simulink model "TV_2018_HIL"  (R2016a)
settings: Solver=FixedStepAuto  StartTime=0.0  StopTime=inf  FixedStep=0.001  RelTol=1e-3
PreLoadFcn:
  | TV_2017_parameters
values from neighbouring files (symbols this model uses):
  battery_voltage = single(530)    [HIL_parameters.m]    (also in HIL_parameters_2018.m; TV_2017_parameters.m; TV_2017_parameters_VD.m)
  car_params = Simulink_Car_params    [HIL_parameters.m]    (also in HIL_parameters_2018.m; TV_2017_parameters.m; TV_2017_parameters_VD.m)
  i_Diff = 16    [HIL_parameters.m]    (also in HIL_parameters_2018.m; TV_2017_parameters.m)
  Kp = 1    [HIL_parameters.m]    (also in HIL_parameters_2018.m; TV_2017_parameters.m; TV_2017_parameters_VD.m)
  motor_data = struct    [HIL_parameters.m]    (also in HIL_parameters_2018.m; TV_2017_parameters.m)
  powerLimitControl = Simulink_el    [HIL_parameters.m]    (also in HIL_parameters_2018.m; TV_2017_parameters.m; TV_2017_parameters_VD.m)
  settings = Simulink_Settings    [HIL_parameters.m]    (also in HIL_parameters_2018.m; TV_2017_parameters.m; TV_2017_parameters_VD.m)
  SpdC_BCC = 0    [HIL_parameters.m]    (also in HIL_parameters_2018.m; TV_2017_parameters.m; TV_2017_parameters_VD.m)
  Speed_Neg_sat = -21    [HIL_parameters.m]    (also in HIL_parameters_2018.m; TV_2017_parameters.m; TV_2017_parameters_VD.m)
  Speed_Pos_sat = 21    [HIL_parameters.m]    (also in HIL_parameters_2018.m; TV_2017_parameters.m; TV_2017_parameters_VD.m)
  SteeringAngleFL = [-23.80 -22.65 -21.50 -20.34 -19.18 -18.03 -16.86 -15.70 -14.53 -13.35 -12.18 -10.99 -9.80 -8.61 -7.40 -6.19 -4.97 -3.75 -2.51 -1.26 0 1.27 2.56 3.85 5.17 6.50 7.84 9.21 10.59 12.00 13.42 14.88 16.36 17.87 19.41 20.99 22.61 24.26 25.97 27.73 29.54]    [CarSetupAnalysis2018.m]    (also in HIL_parameters_2018.m; TV_2017_parameters.m; TV_2017_parameters_VD.m = [-24.129 -22.950 -21.772 -20.593 -19.413 -18.232 -17.050 -15)
  SteeringAngleFR = [-29.54 -27.73 -25.97 -24.26 -22.61 -20.99 -19.41 -17.87 -16.36 -14.88 -13.42 -12.00 -10.59 -9.21 -7.84 -6.50 -5.17 -3.85 -2.56 -1.27 0 1.26 2.51 3.75 4.97 6.19 7.40 8.61 9.80 10.99 12.18 13.35 14.53 15.70 16.86 18.03 19.18 20.34 21.50 22.65 23.80]    [CarSetupAnalysis2018.m]    (also in HIL_parameters_2018.m; TV_2017_parameters.m; TV_2017_parameters_VD.m = [-29.3050 -27.5340 -25.8140 -24.1410 -22.5110 -20.9180 -19.3)
  SteeringWhAngle = [-105 -99.75 -94.5 -89.25 -84 -78.75 -73.5 -68.25 -63 -57.75 -52.5 -47.25 -42 -36.75 -31.5 -26.25 -21.0 -15.75 -10.5 -5.25 0.0 5.25 10.50 15.75 21.00 26.25 31.50 36.75 42.00 47.25 52.50 57.75  63.00 68.25 73.50 78.75 84.00 89.25 94.50 99.75 105.00]    [TV_2017_parameters_VD.m]
  Tn_n = 0    [HIL_parameters.m]    (also in HIL_parameters_2018.m; TV_2017_parameters.m; TV_2017_parameters_VD.m)
  tractionControl = Simulink_tc    [HIL_parameters.m]    (also in HIL_parameters_2018.m; IterativeTractionControlTuning.m; TV_2017_parameters.m; TV_2017_parameters_VD.m)
  yawMomentGenerator = struct    [HIL_parameters.m]    (also in HIL_parameters_2018.m = Simulink_yawRate2; TV_2017_parameters.m = Simulink_yawRate2)
  yawRateControl = Simulink_yawRate    [HIL_parameters.m]    (also in HIL_parameters_2018.m; TV_2017_parameters.m; TV_2017_parameters_VD.m)
undefined symbols (not defined in the file or in its folder): canChannel, DiscIntNeverNeededParam, magnitude, speedEstimation, TC_Decr_Gas, TC_Derivative, TC_Incr_Gas, TC_On, TC_Relay_Off, TC_Relay_On
libraries: CarMaker4SL x366, simulink_extras x63, canmsglib x55, canlib x41, simulink x37, dspfdesign x2, sldrtlib x1
(part 8 of 15)

== system TV_2018_HIL/CarMaker/Subsystem/Control_System /Subsystem/2016 adapted ==
  note: This needs more thought
  Mz_ref : Inport
  T_req : Inport  Port=2
  "States " : Inport  Port=3
  Bus Selector : BusSelector  OutputSignals=mmt_FL,mmt_FR,mmt_RL,mmt_RR
  Constant{1..4} (4 alike) : Constant  Value=int8(0)
  Inverter temperature limiter : MATLAB Function  TreatAsAtomicUnit=on
  MATLAB Function : MATLAB Function  Commented=on  TreatAsAtomicUnit=on
  Motor temperature limiter : MATLAB Function  TreatAsAtomicUnit=on
  Mux18 : Mux
  Mux2 : Mux
  Torque Allocation : Subsystem
  "max combined tire torque based on (Fz, SA,mu) " : MATLAB Function  TreatAsAtomicUnit=on
  "max long tire torque based on (FZ , mu)" : MATLAB Function  TreatAsAtomicUnit=on
  "max torque " : MATLAB Function  TreatAsAtomicUnit=on
  maxMotorTorque and kers based on available power : MATLAB Function  TreatAsAtomicUnit=on
  maxmotortoruq : Scope
  "Mz_allocated " : Outport
  Ti_lim : Outport  Port=2
  saturated_constraints : Outport  Port=3
  Max_motor_torque : Outport  Port=4
  active_constraints : Outport  Port=5
  wires:
  "States "/1 -> [states], Torque Allocation/2(states)
  Mz_ref/1 -> Torque Allocation/4(Mz_ref)
  Bus Selector/1 -> Mux18/1  "<mmt_FL>"
  Bus Selector/2 -> Mux18/2  "<mmt_FR>"
  Bus Selector/3 -> Mux18/3  "<mmt_RL>"
  Bus Selector/4 -> Mux18/4  "<mmt_RR>"
  T_req/1 -> Torque Allocation/1(T_req)
  Torque Allocation/1(Ti_lim) -> Ti_lim/1
  Mux18/1 -> maxmotortoruq/1
  [states] -> maxMotorTorque and kers based on available power/1(states)
  Inverter temperature limiter/1(maxMotorTorque) -> "max torque "/1(calc_pow_lim), "max torque "/2(inv_temp_lim)
  "max torque "/1(maxMotorTorque) -> Max_motor_torque/1, Bus Selector/1, [maxMotorTorque]
  "max torque "/2(active_constraints) -> active_constraints/1, [active_constraints]
  [states] -> Inverter temperature limiter/1(states)
  Motor temperature limiter/1(maxMotorTorque) -> "max torque "/3(mot_temp_lim)
  [states] -> Motor temperature limiter/1(states)
  "max long tire torque based on (FZ , mu)"/1(maxMotorTorque) -> "max torque "/5(SA_lim), "max torque "/4(mu_lim)
  [states] -> "max long tire torque based on (FZ , mu)"/1(states)
  "max combined tire torque based on (Fz, SA,mu) "/1(maxMotorTorque) -> ?
  [states] -> "max combined tire torque based on (Fz, SA,mu) "/1(states)
  maxMotorTorque and kers based on available power/1(maxMotorTorque) -> ?
  Mux2/1 -> saturated_constraints/1
  Constant1/1 -> Mux2/1  "<mmt_FL>"
  Constant2/1 -> Mux2/2  "<mmt_FR>"
  Constant3/1 -> Mux2/3  "<mmt_RL>"
  Constant4/1 -> Mux2/4  "<mmt_RR>"
  Torque Allocation/2(Mz_allocated) -> "Mz_allocated "/1
  [maxMotorTorque] -> Torque Allocation/3(maxMotorTorque)

== system TV_2018_HIL/CarMaker/Subsystem/Control_System /Subsystem/Torque allocation 2016 ==
  Mz_ref : Inport
  T_req : Inport  Port=2
  "States " : Inport  Port=3
  Bus Selector : BusSelector  OutputSignals=mmt_FL,mmt_FR,mmt_RL,mmt_RR
  MATLAB Function : MATLAB Function  TreatAsAtomicUnit=on
  Mux18 : Mux
  Torque Allocation : Subsystem
  maxmotortoruq : Scope
  Ti_lim : Outport
  "Mz_error " : Outport  Port=2
  Max_motor_torque_i : Outport  Port=3
  wires:
  "States "/1 -> MATLAB Function/1(states), Torque Allocation/2(states)
  Mz_ref/1 -> Torque Allocation/4(Mz_ref)
  Torque Allocation/2(Mz_error) -> "Mz_error "/1
  MATLAB Function/1(maxMotorTorque) -> Bus Selector/1, Torque Allocation/3(maxMotorTorque)
  Bus Selector/1 -> Mux18/1  "<mmt_FL>"
  Bus Selector/2 -> Mux18/2  "<mmt_FR>"
  Bus Selector/3 -> Mux18/3  "<mmt_RL>"
  Bus Selector/4 -> Mux18/4  "<mmt_RR>"
  T_req/1 -> Torque Allocation/1(T_req)
  Torque Allocation/1(Ti_lim) -> Ti_lim/1
  Mux18/1 -> Max_motor_torque_i/1, maxmotortoruq/1

== system TV_2018_HIL/CarMaker/Subsystem/Control_System /Subsystem/Torque allocation 2017 ==
  Mz_ref : Inport
  T_req : Inport  Port=2
  "States " : Inport  Port=3
  Bus Creator : BusCreator  Commented=on  Inputs=2  OutDataTypeStr=Bus: maxMotorTorque
  Bus Selector1 : BusSelector  Commented=on  OutputSignals=mmt_FL,mmt_FR,mmt_RL,mmt_RR
  Constant{1..4} (4 alike) : Constant  Value=int8(1)
  Inverter temperature limiter : MATLAB Function  TreatAsAtomicUnit=on
  Motor temperature limiter : MATLAB Function  TreatAsAtomicUnit=on
  Mux2 : Mux
  Scope : Scope
  Scope1 : Scope  Commented=on  NumInputPorts=4
  Torque Allocation Quadratic Programming : MATLAB Function  TreatAsAtomicUnit=on
  "max combined tire torque based on (Fz, SA,mu) " : MATLAB Function  TreatAsAtomicUnit=on
  "max long tire torque based on (FZ , mu)" : MATLAB Function  TreatAsAtomicUnit=on
  "max torque " : MATLAB Function  TreatAsAtomicUnit=on
  maxMotorTorque and kers based on available power : MATLAB Function  TreatAsAtomicUnit=on
  "Mz_allocated " : Outport
  Ti_lim : Outport  Port=2
  saturated_constraints : Outport  Port=3
  max_motor_torque : Outport  Port=4
  active_constraints : Outport  Port=5
  wires:
  [states] -> maxMotorTorque and kers based on available power/1(states)
  "max torque "/2(active_constraints) -> [active_constraints]
  [states] -> Inverter temperature limiter/1(states)
  Motor temperature limiter/1(maxMotorTorque) -> "max torque "/4(mot_temp_lim)
  [states] -> Motor temperature limiter/1(states)
  "max long tire torque based on (FZ , mu)"/1(maxMotorTorque) -> "max torque "/2(SA_lim), "max torque "/1(mu_lim)
  [states] -> "max long tire torque based on (FZ , mu)"/1(states)
  [states] -> "max combined tire torque based on (Fz, SA,mu) "/1(states)
  [maxMotorTorque] -> max_motor_torque/1
  [active_constraints] -> active_constraints/1
  Mux2/1 -> saturated_constraints/1
  Constant1/1 -> Mux2/1  "<mmt_FL>"
  Constant2/1 -> Mux2/2  "<mmt_FR>"
  Constant3/1 -> Mux2/3  "<mmt_RL>"
  Constant4/1 -> Mux2/4  "<mmt_RR>"
  Mz_ref/1 -> ?  "Mz_ref"
  T_req/1 -> ?
  "States "/1 -> [states]
  [states] -> ?
  [maxMotorTorque] -> ?
  ? -> Ti_lim/1
  ? -> "Mz_allocated "/1
  "max torque "/1(maxMotorTorque) -> Bus Selector1/1, [maxMotorTorque]
  Bus Selector1/1 -> Scope1/1  "<mmt_FL>"
  Bus Selector1/2 -> Scope1/2  "<mmt_FR>"
  Bus Selector1/3 -> Scope1/3  "<mmt_RL>"
  Bus Selector1/4 -> Scope1/4  "<mmt_RR>"
  Inverter temperature limiter/1(maxMotorTorque) -> "max torque "/3(inv_temp_lim)
  "max combined tire torque based on (Fz, SA,mu) "/1(maxMotorTorque) -> ?

== system TV_2018_HIL/CarMaker/Subsystem/Control_System /Subsystem/Torque allocation QP- ==
  Mz_ref : Inport
  T_req : Inport  Port=2
  "States " : Inport  Port=3
  Bus Creator : BusCreator  Commented=on  Inputs=2  OutDataTypeStr=Bus: maxMotorTorque
  Bus Selector1 : BusSelector  OutputSignals=mmt_FL,mmt_FR,mmt_RL,mmt_RR
  Constant{1..4} (4 alike) : Constant  Value=int8(1)
  Inverter temperature limiter : MATLAB Function  TreatAsAtomicUnit=on
  Motor temperature limiter : MATLAB Function  TreatAsAtomicUnit=on
  Mux2 : Mux
  Scope : Scope
  Scope1 : Scope  NumInputPorts=4
  Torque Allocation Quadratic Programming : MATLAB Function  TreatAsAtomicUnit=on
  "max combined tire torque based on (Fz, SA,mu) " : MATLAB Function  TreatAsAtomicUnit=on
  "max long tire torque based on (FZ , mu)" : MATLAB Function  TreatAsAtomicUnit=on
  "max torque " : MATLAB Function  TreatAsAtomicUnit=on
  maxMotorTorque and kers based on available power : MATLAB Function  TreatAsAtomicUnit=on
  "Mz_allocated " : Outport
  Ti_lim : Outport  Port=2
  saturated_constraints : Outport  Port=3
  max_motor_torque : Outport  Port=4
  active_constraints : Outport  Port=5
  wires:
  [states] -> maxMotorTorque and kers based on available power/1(states)
  "max torque "/2(active_constraints) -> [active_constraints]
  [states] -> Inverter temperature limiter/1(states)
  Motor temperature limiter/1(maxMotorTorque) -> "max torque "/4(mot_temp_lim)
  [states] -> Motor temperature limiter/1(states)
  "max long tire torque based on (FZ , mu)"/1(maxMotorTorque) -> "max torque "/2(SA_lim), "max torque "/1(mu_lim)
  [states] -> "max long tire torque based on (FZ , mu)"/1(states)
  [states] -> "max combined tire torque based on (Fz, SA,mu) "/1(states)
  [maxMotorTorque] -> max_motor_torque/1
  [active_constraints] -> active_constraints/1
  Mux2/1 -> saturated_constraints/1
  Constant1/1 -> Mux2/1  "<mmt_FL>"
  Constant2/1 -> Mux2/2  "<mmt_FR>"
  Constant3/1 -> Mux2/3  "<mmt_RL>"
  Constant4/1 -> Mux2/4  "<mmt_RR>"
  Mz_ref/1 -> Torque Allocation Quadratic Programming/1(Mz_ref)  "Mz_ref"
  T_req/1 -> Torque Allocation Quadratic Programming/2(T_req)
  "States "/1 -> [states]
  [states] -> Torque Allocation Quadratic Programming/3(states)
  [maxMotorTorque] -> Torque Allocation Quadratic Programming/4(maxMotorTorque)
  Torque Allocation Quadratic Programming/1(Ti_lim) -> Ti_lim/1
  Torque Allocation Quadratic Programming/3(Mz_allocated) -> "Mz_allocated "/1
  "max torque "/1(maxMotorTorque) -> Bus Selector1/1, [maxMotorTorque]
  Bus Selector1/1 -> Scope1/1  "<mmt_FL>"
  Bus Selector1/2 -> Scope1/2  "<mmt_FR>"
  Bus Selector1/3 -> Scope1/3  "<mmt_RL>"
  Bus Selector1/4 -> Scope1/4  "<mmt_RR>"
  Inverter temperature limiter/1(maxMotorTorque) -> "max torque "/3(inv_temp_lim)

== system TV_2018_HIL/CarMaker/Subsystem/Control_System /Subsystem/Torque allocation QP-1 ==
  Mz_ref : Inport
  T_req : Inport  Port=2
  "States " : Inport  Port=3
  Bus Creator : BusCreator  Commented=on  Inputs=2  OutDataTypeStr=Bus: maxMotorTorque
  Bus Selector1 : BusSelector  OutputSignals=mmt_FL,mmt_FR,mmt_RL,mmt_RR
  Constant{1..4} (4 alike) : Constant  Value=int8(1)
  Inverter temperature limiter : MATLAB Function  TreatAsAtomicUnit=on
  Motor temperature limiter : MATLAB Function  TreatAsAtomicUnit=on
  Mux2 : Mux
  Scope : Scope
  Scope1 : Scope  NumInputPorts=4
  Torque Allocation Quadratic Programming : MATLAB Function  TreatAsAtomicUnit=on
  "max combined tire torque based on (Fz, SA,mu) " : MATLAB Function  TreatAsAtomicUnit=on
  "max long tire torque based on (FZ , mu)" : MATLAB Function  TreatAsAtomicUnit=on
  "max torque " : MATLAB Function  TreatAsAtomicUnit=on
  maxMotorTorque and kers based on available power : MATLAB Function  TreatAsAtomicUnit=on
  "Mz_allocated " : Outport
  Ti_lim : Outport  Port=2
  saturated_constraints : Outport  Port=3
  max_motor_torque : Outport  Port=4
  active_constraints : Outport  Port=5
  wires:
  [states] -> maxMotorTorque and kers based on available power/1(states)
  "max torque "/2(active_constraints) -> [active_constraints]
  [states] -> Inverter temperature limiter/1(states)
  Motor temperature limiter/1(maxMotorTorque) -> "max torque "/4(mot_temp_lim)
  [states] -> Motor temperature limiter/1(states)
  "max long tire torque based on (FZ , mu)"/1(maxMotorTorque) -> "max torque "/2(SA_lim), "max torque "/1(mu_lim)
  [states] -> "max long tire torque based on (FZ , mu)"/1(states)
  [states] -> "max combined tire torque based on (Fz, SA,mu) "/1(states)
  [maxMotorTorque] -> max_motor_torque/1
  [active_constraints] -> active_constraints/1
  Mux2/1 -> saturated_constraints/1
  Constant1/1 -> Mux2/1  "<mmt_FL>"
  Constant2/1 -> Mux2/2  "<mmt_FR>"
  Constant3/1 -> Mux2/3  "<mmt_RL>"
  Constant4/1 -> Mux2/4  "<mmt_RR>"
  Mz_ref/1 -> Torque Allocation Quadratic Programming/1(Mz_ref)  "Mz_ref"
  T_req/1 -> Torque Allocation Quadratic Programming/2(T_req)
  "States "/1 -> [states]
  [states] -> Torque Allocation Quadratic Programming/3(states)
  [maxMotorTorque] -> Torque Allocation Quadratic Programming/4(maxMotorTorque)
  Torque Allocation Quadratic Programming/1(Ti_lim) -> Ti_lim/1
  Torque Allocation Quadratic Programming/3(Mz_allocated) -> "Mz_allocated "/1
  "max torque "/1(maxMotorTorque) -> Bus Selector1/1, [maxMotorTorque]
  Bus Selector1/1 -> Scope1/1  "<mmt_FL>"
  Bus Selector1/2 -> Scope1/2  "<mmt_FR>"
  Bus Selector1/3 -> Scope1/3  "<mmt_RL>"
  Bus Selector1/4 -> Scope1/4  "<mmt_RR>"
  Inverter temperature limiter/1(maxMotorTorque) -> "max torque "/3(inv_temp_lim)

== system TV_2018_HIL/CarMaker/Subsystem/Control_System /TA 2017/Slip handling (Traction Control)  ==
  Sensors : Inport
  Memory : Memory  InheritSampleTime=on
  Memory1 : Memory  InheritSampleTime=on
  Scaling factors from slip detection : MATLAB Function  TreatAsAtomicUnit=on
  slipScalingFactors : Outport
  wires:
  Sensors/1 -> Scaling factors from slip detection/1(states)
  Scaling factors from slip detection/2(duration) -> Memory1/1
  Memory/1 -> Scaling factors from slip detection/3(prev_slip)
  Scaling factors from slip detection/3(slip) -> Memory/1
  Memory1/1 -> Scaling factors from slip detection/2(prev_duration)
  Scaling factors from slip detection/1(slipScalingFactor) -> slipScalingFactors/1

== system TV_2018_HIL/CarMaker/Subsystem/Control_System /Yaw_rate_Mz_generator/Yaw Rate Controller  ==
  "Mz_error " : Inport
  States : Inport  Port=2
  Data Type Conversion : DataTypeConversion  OutDataTypeStr=single  RndMeth=Round
  Discrete-Time Integrator2 : DiscreteIntegrator  InitialConditionSetting=State (most efficient)  SampleTime=-1  LimitOutput=on  UpperSaturationLimit=yawRateControl.max_moment  LowerSaturationLimit=-yawRateControl.max_moment  ICPrevOutput=DiscIntNeverNeededParam  ICPrevScaledInput=DiscIntNeverNeededParam
  Enable/disable : Constant  Value=yawRateControl.enable
  Gain1 : Gain  Gain=single(3.6)
  Ksat : Constant  Value=yawRateControl.Ksat
  Memory : Memory  InheritSampleTime=on
  Mz_ref_YRR : Scope  NumInputPorts=2
  "Mzerror " : Scope
  Mzerror 1 : Scope  NumInputPorts=2
  PI_Ki 3 : Scope
  Product{7..8,10..11} (4 alike) : Product
  Product3 : Product  OutDataTypeStr=single
  Saturation : Saturate  UpperLimit=yawRateControl.max_moment  LowerLimit=-yawRateControl.max_moment
  Sum2 : Sum  Inputs=+++  AccumDataTypeStr=single
  Sum3 : Sum  Inputs=|+-
  gainScheduling : MATLAB Function  TreatAsAtomicUnit=on
  "not NaN " : MATLAB Function  TreatAsAtomicUnit=on
  not not a number : MATLAB Function  TreatAsAtomicUnit=on
  yawRateReference : MATLAB Function  TreatAsAtomicUnit=on
  "r_ref " : Outport
  r_lim : Outport  Port=2
  Mz_ref : Outport  Port=3  OutDataTypeStr=single
  Mz_ref_to_telemetry : Outport  Port=4  OutDataTypeStr=single
  wires:
  States/1 -> yawRateReference/1(states)
  yawRateReference/4(r_ref) -> "r_ref "/1
  yawRateReference/5(r_lim) -> r_lim/1
  Product7/1 -> Sum2/2
  Sum2/1 -> Mz_ref_to_telemetry/1, Product3/2
  Product8/1 -> Sum3/1
  Sum3/1 -> Discrete-Time Integrator2/1
  Discrete-Time Integrator2/1 -> PI_Ki 3/1, Sum2/3
  Product11/1 -> not not a number/1(in)
  yawRateReference/1(r_der_error) -> Product10/1
  Product10/1 -> Sum2/1
  gainScheduling/2(Kp) -> Mzerror 1/1, Product7/1
  Ksat/1 -> Product11/1
  "Mz_error "/1 -> "Mzerror "/1, Product11/2
  gainScheduling/3(Ki) -> Product8/1, Mzerror 1/2
  yawRateReference/2(r_error) -> Memory/1, Product8/2, Product7/2
  Product3/1 -> Saturation/1
  Enable/disable/1 -> Product3/1
  yawRateReference/3(vx) -> Gain1/1
  Gain1/1 -> gainScheduling/1(vx_kmh)
  gainScheduling/1(Kd) -> Product10/2
  not not a number/1(out) -> Sum3/2
  Saturation/1 -> "not NaN "/1(in)
  "not NaN "/1(out) -> Data Type Conversion/1, Mz_ref_YRR/1
  Data Type Conversion/1 -> Mz_ref_YRR/2, Mz_ref/1
  Memory/1 -> yawRateReference/2(prev_r_error)

== system TV_2018_HIL/CarMaker/Subsystem/Control_System /Yaw_rate_Mz_generator/Yaw Rate Generator ==
  States : Inport
  Yaw Rate ref : Scope  NumInputPorts=3
  yawRateGenerator : MATLAB Function  TreatAsAtomicUnit=on
  Mz_ref : Outport  OutDataTypeStr=single
  Mz_ref_to_telemetry : Outport  Port=2  OutDataTypeStr=single
  wires:
  yawRateGenerator/1(Mz_ref) -> Yaw Rate ref/1, Mz_ref/1
  States/1 -> yawRateGenerator/1(states)
  yawRateGenerator/3(Kp_term) -> Yaw Rate ref/2
  yawRateGenerator/4(Kd_term) -> Yaw Rate ref/3
  yawRateGenerator/2(Mz_ref_to_telemetry) -> Mz_ref_to_telemetry/1

== system TV_2018_HIL/CarMaker/Subsystem/Estimations/Fz_estimators/Fz_Estimation ==
  sensors : Inport
  1st_deriv : Subsystem
  2nd_deriv : Subsystem
  Bus Selector : BusSelector  OutputSignals=damper_rate_FL,damper_rate_FR,damper_rate_RL,damper_rate_RR
  Bus Selector1 : BusSelector  OutputSignals=FL,FR,RL,RR
  DamperRateLookup : Lookup_n-D  NumberOfTableDimensions=1  BreakpointsForDimension1=car_params.damper_table_breakpoint;  Table=car_params.damper_pull_push_values_front;  ExtrapMethod=Clip  UseLastTableValue=on  InternalRulePriority=Speed  RndMeth=Simplest  InputSameDT=on
  DamperRateLookup1 : Lookup_n-D  NumberOfTableDimensions=1  BreakpointsForDimension1=car_params.damper_table_breakpoint;  Table=car_params.damper_pull_push_values_front;  ExtrapMethod=Clip  UseLastTableValue=on  InternalRulePriority=Speed  RndMeth=Simplest  InputSameDT=on
  DamperRateLookup2 : Lookup_n-D  NumberOfTableDimensions=1  BreakpointsForDimension1=car_params.damper_table_breakpoint;  Table=car_params.damper_pull_push_values_rear;  ExtrapMethod=Clip  UseLastTableValue=on  InternalRulePriority=Speed  RndMeth=Simplest  InputSameDT=on
  DamperRateLookup3 : Lookup_n-D  NumberOfTableDimensions=1  BreakpointsForDimension1=car_params.damper_table_breakpoint;  Table=car_params.damper_pull_push_values_rear;  ExtrapMethod=Clip  UseLastTableValue=on  InternalRulePriority=Speed  RndMeth=Simplest  InputSameDT=on
  FZ_etsimate : Scope  NumInputPorts=4
  FzEstDamper : MATLAB Function  TreatAsAtomicUnit=on
  Scope2 : Scope  NumInputPorts=4
  Sum : Sum  Inputs=|++++
  Sum_FZ : Scope
  alfa_r_scope : Scope
  Fz_est : Outport
  alfa_r : Outport  Port=2
  wires:
  sensors/1 -> FzEstDamper/1(sensors), Bus Selector/1
  Bus Selector/1 -> DamperRateLookup/1  "<damper_rate_FL>"
  Bus Selector/2 -> DamperRateLookup1/1  "<damper_rate_FR>"
  Bus Selector/3 -> DamperRateLookup2/1  "<damper_rate_RL>"
  Bus Selector/4 -> DamperRateLookup3/1  "<damper_rate_RR>"
  FzEstDamper/2(alfa_r) -> alfa_r_scope/1, alfa_r/1
  Bus Selector1/2 -> Sum/3, FZ_etsimate/2  "<FR>"
  Bus Selector1/1 -> Sum/4, FZ_etsimate/1  "<FL>"
  Bus Selector1/3 -> Sum/2, FZ_etsimate/3  "<RL>"
  Bus Selector1/4 -> FZ_etsimate/4, Sum/1  "<RR>"
  FzEstDamper/1(Fz_damper_est) -> Bus Selector1/1, Fz_est/1
  DamperRateLookup1/1 -> Scope2/2, FzEstDamper/3(Fz_damp_FR)  "<FR>"
  DamperRateLookup/1 -> Scope2/1, FzEstDamper/2(Fz_damp_FL)  "<FL>"
  DamperRateLookup2/1 -> Scope2/3, FzEstDamper/4(Fz_damp_RL)  "<RL>"
  DamperRateLookup3/1 -> Scope2/4, FzEstDamper/5(Fz_damp_RR)  "<RR>"
  Sum/1 -> Sum_FZ/1

== system TV_2018_HIL/CarMaker/Subsystem/Estimations/Fz_estimators/Fz_Estimation_acceleration based ==
  sensors : Inport
  Bus Selector1 : BusSelector  OutputSignals=FL,FR,RL,RR
  Bus Selector2 : BusSelector  OutputSignals=Input_throttle,Input_brake,KERS_pos
  FZ_etsimate_acceleration : Scope  NumInputPorts=4
  Fz_acc_est : MATLAB Function  TreatAsAtomicUnit=on
  Lowpass Filter : dspfdesign/Lowpass Filter  FilterType=FIR  DesignForMinimumOrder=on  FilterOrder=50  PassbandFrequency=4  StopbandFrequency=15  PassbandRipple=0.1  StopbandAttenuation=80  InheritSampleRate=on  SampleRate=100  roundingMode=Floor  coeffsDataTypeStr=fixdt(1,16)  SimulateUsing=Interpreted execution
  Lowpass Filter1 : dspfdesign/Lowpass Filter  FilterType=FIR  DesignForMinimumOrder=on  FilterOrder=50  PassbandFrequency=4  StopbandFrequency=15  PassbandRipple=0.1  StopbandAttenuation=80  InheritSampleRate=on  SampleRate=100  roundingMode=Floor  coeffsDataTypeStr=fixdt(1,16)  SimulateUsing=Code generation
  alfa_r_acc : Scope  NumInputPorts=2
  alfa_r_acc_tps_bps_kers : Scope  NumInputPorts=4
  filtervsUnfilter : Scope  NumInputPorts=2
  "Fz_acc " : Outport
  "alfa_r_acc " : Outport  Port=2
  wires:
  sensors/1 -> Bus Selector2/1, Fz_acc_est/1(sensors)
  Bus Selector1/2 -> FZ_etsimate_acceleration/2  "<FR>"
  Bus Selector1/1 -> Lowpass Filter/1, filtervsUnfilter/2, FZ_etsimate_acceleration/1  "<FL>"
  Bus Selector1/3 -> FZ_etsimate_acceleration/3  "<RL>"
  Bus Selector1/4 -> FZ_etsimate_acceleration/4  "<RR>"
  Fz_acc_est/1(Fz_acc_est) -> "Fz_acc "/1, Bus Selector1/1
  Lowpass Filter/1 -> filtervsUnfilter/1
  Lowpass Filter1/1 -> alfa_r_acc/1
  Fz_acc_est/2(alfa_r_acc) -> alfa_r_acc_tps_bps_kers/1, "alfa_r_acc "/1, alfa_r_acc/2, Lowpass Filter1/1
  Bus Selector2/1 -> alfa_r_acc_tps_bps_kers/2  "<Input_throttle>"
  Bus Selector2/2 -> alfa_r_acc_tps_bps_kers/3  "<Input_brake>"
  Bus Selector2/3 -> alfa_r_acc_tps_bps_kers/4  "<KERS_pos>"

== system TV_2018_HIL/CarMaker/Subsystem/Estimations/Subsystem/SA calculation ==
  sensor : Inport
  Bus Selector2 : BusSelector  OutputSignals=steering_wheel_angle
  Degrees to Radians : simulink_extras/Transformations/Degrees to Radians
  Degrees to Radians1 : simulink_extras/Transformations/Degrees to Radians
  FL steer ang lookup deg : Lookup_n-D  NumberOfTableDimensions=1  BreakpointsForDimension1=SteeringAngleFL  Table=SteeringAngleFL  ExtrapMethod=Clip  UseLastTableValue=on  InternalRulePriority=Speed  RndMeth=Simplest  InputSameDT=on
  FR steer ang lookup deg : Lookup_n-D  NumberOfTableDimensions=1  BreakpointsForDimension1=SteeringAngleFR  Table=SteeringAngleFR  ExtrapMethod=Clip  UseLastTableValue=on  InternalRulePriority=Speed  RndMeth=Simplest  InputSameDT=on
  Radians to Degrees1 : simulink_extras/Transformations/Radians to Degrees
  Slip angle calc : MATLAB Function  Commented=on  TreatAsAtomicUnit=on
  Slip angle calc1 : MATLAB Function  TreatAsAtomicUnit=on
  SA : Outport
  wires:
  Radians to Degrees1/1 -> FL steer ang lookup deg/1, FR steer ang lookup deg/1
  Degrees to Radians1/1 -> Slip angle calc1/2(wheel_ang_right)
  Slip angle calc1/1(SA) -> SA/1
  FR steer ang lookup deg/1 -> Degrees to Radians1/1
  sensor/1 -> Slip angle calc1/3(sensor), Bus Selector2/1
  FL steer ang lookup deg/1 -> Degrees to Radians/1
  Bus Selector2/1 -> Radians to Degrees1/1  "<steering_wheel_angle>"
  Degrees to Radians/1 -> Slip angle calc1/1(wheel_ang_left)

== system TV_2018_HIL/CarMaker/Subsystem/Estimations/Subsystem/SR_Calculation ==
  v_x : Inport
  whl_v : Inport  Port=2
  sensorInput : Inport  Port=3
  Slip ratio : MATLAB Function  TreatAsAtomicUnit=on
  SR : Outport
  wires:
  v_x/1 -> Slip ratio/1(V_x)
  Slip ratio/1(SR) -> SR/1
  whl_v/1 -> Slip ratio/2(whl_v)
  sensorInput/1 -> Slip ratio/3(sensor)

== system TV_2018_HIL/CarMaker/Subsystem/Estimations/Subsystem/Slip_Detection ==
  sensor : Inport
  SR : Inport  Port=2
  Memory : Memory  InheritSampleTime=on
  Slip Detection : MATLAB Function  TreatAsAtomicUnit=on
  slip : Outport
  wires:
  Slip Detection/1(slip) -> Memory/1, slip/1
  SR/1 -> Slip Detection/1(SR)
  sensor/1 -> Slip Detection/2(sensors)
  Memory/1 -> Slip Detection/3(slip_prev)

== system TV_2018_HIL/CarMaker/IPG Vehicle3/CarAndTrailer/Forces/Tires/TireFL ==
  note: Insert your tire model here.
  Sync_In : Inport
  Load : Inport  Port=2
  vxtrans : Inport  Port=3
  vytrans : Inport  Port=4
  Rim_rotv : Inport  Port=5
  Rim_turnv : Inport  Port=6
  InclinAngle : Inport  Port=7
  muRoad : Inport  Port=8
  Ground{1..11} (11 alike) : Ground
  Terminator{,1..6,12} (8 alike) : Terminator
  Slp : Outport
  Alpha : Outport  Port=2
  TurnSlp : Outport  Port=3
  rBelt_eff : Outport  Port=4
  vBelt : Outport  Port=5
  LongFrc : Outport  Port=6
  SideFrc : Outport  Port=7
  LoadFrc : Outport  Port=8
  OverturnTrq : Outport  Port=9
  RollResist : Outport  Port=10
  AlignTrq : Outport  Port=11
  wires:
  Ground11/1 -> vBelt/1
  Ground10/1 -> rBelt_eff/1
  Ground9/1 -> TurnSlp/1
  Rim_turnv/1 -> Terminator6/1
  Sync_In/1 -> Terminator12/1
  Ground2/1 -> Alpha/1
  Ground3/1 -> LongFrc/1
  Ground4/1 -> SideFrc/1
  Ground5/1 -> OverturnTrq/1
  vxtrans/1 -> Terminator1/1
  vytrans/1 -> Terminator2/1
  Rim_rotv/1 -> Terminator3/1
  InclinAngle/1 -> Terminator4/1
  muRoad/1 -> Terminator5/1
  Load/1 -> Terminator/1
  Ground1/1 -> Slp/1
  Ground6/1 -> LoadFrc/1
  Ground7/1 -> RollResist/1
  Ground8/1 -> AlignTrq/1

== system TV_2018_HIL/CarMaker/IPG Vehicle3/CarAndTrailer/Forces/Tires/TireFR ==
  note: Insert your tire model here.
  Sync_In : Inport
  Load : Inport  Port=2
  vxtrans : Inport  Port=3
  vytrans : Inport  Port=4
  Rim_rotv : Inport  Port=5
  Rim_turnv : Inport  Port=6
  InclinAngle : Inport  Port=7
  muRoad : Inport  Port=8
  Ground{1..11} (11 alike) : Ground
  Terminator{,1..6,12} (8 alike) : Terminator
  Slp : Outport
  Alpha : Outport  Port=2
  TurnSlp : Outport  Port=3
  rBelt_eff : Outport  Port=4
  vBelt : Outport  Port=5
  LongFrc : Outport  Port=6
  SideFrc : Outport  Port=7
  LoadFrc : Outport  Port=8
  OverturnTrq : Outport  Port=9
  RollResist : Outport  Port=10
  AlignTrq : Outport  Port=11
  wires:
  Ground11/1 -> vBelt/1
  Ground10/1 -> rBelt_eff/1
  Ground9/1 -> TurnSlp/1
  Rim_turnv/1 -> Terminator6/1
  Sync_In/1 -> Terminator12/1
  Ground2/1 -> Alpha/1
  Ground3/1 -> LongFrc/1
  Ground4/1 -> SideFrc/1
  Ground5/1 -> OverturnTrq/1
  vxtrans/1 -> Terminator1/1
  vytrans/1 -> Terminator2/1
  Rim_rotv/1 -> Terminator3/1
  InclinAngle/1 -> Terminator4/1
  muRoad/1 -> Terminator5/1
  Load/1 -> Terminator/1
  Ground1/1 -> Slp/1
  Ground6/1 -> LoadFrc/1
  Ground7/1 -> RollResist/1
  Ground8/1 -> AlignTrq/1

== system TV_2018_HIL/CarMaker/IPG Vehicle3/CarAndTrailer/Forces/Tires/TireRL ==
  note: Insert your tire model here.
  Sync_In : Inport
  Load : Inport  Port=2
  vxtrans : Inport  Port=3
  vytrans : Inport  Port=4
  Rim_rotv : Inport  Port=5
  Rim_turnv : Inport  Port=6
  InclinAngle : Inport  Port=7
  muRoad : Inport  Port=8
  Ground{1..11} (11 alike) : Ground
  Terminator{,1..6,12} (8 alike) : Terminator
  Slp : Outport
  Alpha : Outport  Port=2
  TurnSlp : Outport  Port=3
  rBelt_eff : Outport  Port=4
  vBelt : Outport  Port=5
  LongFrc : Outport  Port=6
  SideFrc : Outport  Port=7
  LoadFrc : Outport  Port=8
  OverturnTrq : Outport  Port=9
  RollResist : Outport  Port=10
  AlignTrq : Outport  Port=11
  wires:
  Ground11/1 -> vBelt/1
  Ground10/1 -> rBelt_eff/1
  Ground9/1 -> TurnSlp/1
  Rim_turnv/1 -> Terminator6/1
  Sync_In/1 -> Terminator12/1
  Ground2/1 -> Alpha/1
  Ground3/1 -> LongFrc/1
  Ground4/1 -> SideFrc/1
  Ground5/1 -> OverturnTrq/1
  vxtrans/1 -> Terminator1/1
  vytrans/1 -> Terminator2/1
  Rim_rotv/1 -> Terminator3/1
  InclinAngle/1 -> Terminator4/1
  muRoad/1 -> Terminator5/1
  Load/1 -> Terminator/1
  Ground1/1 -> Slp/1
  Ground6/1 -> LoadFrc/1
  Ground7/1 -> RollResist/1
  Ground8/1 -> AlignTrq/1

== system TV_2018_HIL/CarMaker/IPG Vehicle3/CarAndTrailer/Forces/Tires/TireRR ==
  note: Insert your tire model here.
  Sync_In : Inport
  Load : Inport  Port=2
  vxtrans : Inport  Port=3
  vytrans : Inport  Port=4
  Rim_rotv : Inport  Port=5
  Rim_turnv : Inport  Port=6
  InclinAngle : Inport  Port=7
  muRoad : Inport  Port=8
  Ground{1..11} (11 alike) : Ground
  Terminator{,1..6,12} (8 alike) : Terminator
  Slp : Outport
  Alpha : Outport  Port=2
  TurnSlp : Outport  Port=3
  rBelt_eff : Outport  Port=4
  vBelt : Outport  Port=5
  LongFrc : Outport  Port=6
  SideFrc : Outport  Port=7
  LoadFrc : Outport  Port=8
  OverturnTrq : Outport  Port=9
  RollResist : Outport  Port=10
  AlignTrq : Outport  Port=11
  wires:
  Ground11/1 -> vBelt/1
  Ground10/1 -> rBelt_eff/1
  Ground9/1 -> TurnSlp/1
  Rim_turnv/1 -> Terminator6/1
  Sync_In/1 -> Terminator12/1
  Ground2/1 -> Alpha/1
  Ground3/1 -> LongFrc/1
  Ground4/1 -> SideFrc/1
  Ground5/1 -> OverturnTrq/1
  vxtrans/1 -> Terminator1/1
  vytrans/1 -> Terminator2/1
  Rim_rotv/1 -> Terminator3/1
  InclinAngle/1 -> Terminator4/1
  muRoad/1 -> Terminator5/1
  Load/1 -> Terminator/1
  Ground1/1 -> Slp/1
  Ground6/1 -> LoadFrc/1
  Ground7/1 -> RollResist/1
  Ground8/1 -> AlignTrq/1

== system TV_2018_HIL/CarMaker/IPG Vehicle3/CarAndTrailer/Forces/Vehicle Forces/Aero R18 prelim ==
  car Aero ApproachVel_1 x : Inport
  car Aero ApproachVel_1 y : Inport  Port=2
  car Aero ApproachVel_1 z : Inport  Port=3
  car Aero tau_1 : Inport  Port=4
  car Aero PoA_1 x : Inport  Port=5
  car Aero PoA_1 y : Inport  Port=6
  car Aero PoA_1 z : Inport  Port=7
  car Aero Frc_1 x : Inport  Port=8
  car Aero Frc_1 y : Inport  Port=9
  car Aero Frc_1 z : Inport  Port=10
  car Aero Trq_1 x : Inport  Port=11
  car Aero Trq_1 y : Inport  Port=12
  car Aero Trq_1 z : Inport  Port=13
  Coefficients : Subsystem
  Constant : Constant  Value=0
  Drag & DF : Scope  NumInputPorts=2
  MATLAB Function : MATLAB Function  TreatAsAtomicUnit=on
  Pitch moment : Scope
  Rad2Deg : simulink_extras/Transformations/Radians to Degrees
  Rad2Deg1 : simulink_extras/Transformations/Radians to Degrees
  Rad2Deg2 : simulink_extras/Transformations/Radians to Degrees
  Read CM Dict : CarMaker4SL/Read CM Dict  xname=Car.Roll  xsync=off
  Read CM Dict1 : CarMaker4SL/Read CM Dict  xname=Car.Pitch  xsync=off
  Read CM Dict2 : CarMaker4SL/Read CM Dict  xname=Car.TrackRadius  xsync=off
  Scope : Scope  Commented=on  NumInputPorts=2
  Terminator{,1..5} (6 alike) : Terminator
  Yaw moment : Scope
  car Aero ApproachVel_1 x_R18 : Outport
  car Aero ApproachVel_1 y_R18 : Outport  Port=2
  car Aero ApproachVel_1 z_R18 : Outport  Port=3
  car Aero tau_1_R18 : Outport  Port=4
  car Aero PoA_1 x_R18 : Outport  Port=5
  car Aero PoA_1 y_R18 : Outport  Port=6
  car Aero PoA_1 z_R18 : Outport  Port=7
  car Aero Frc_1 x_R18 : Outport  Port=8
  car Aero Frc_1 y_R18 : Outport  Port=9
  car Aero Frc_1 z_R18 : Outport  Port=10
  car Aero Trq_1 x_R18 : Outport  Port=11
  car Aero Trq_1 y_R18 : Outport  Port=12
  car Aero Trq_1 z_R18 : Outport  Port=13
  wires:
  Read CM Dict1/1 -> Rad2Deg1/1
  Read CM Dict/1 -> Rad2Deg/1
  car Aero PoA_1 x/1 -> car Aero PoA_1 x_R18/1
  car Aero PoA_1 y/1 -> car Aero PoA_1 y_R18/1
  car Aero PoA_1 z/1 -> car Aero PoA_1 z_R18/1
  Read CM Dict2/1 -> Scope/1, Coefficients/5(Radius)
  Rad2Deg1/1 -> Scope/2, Coefficients/2(Pitch)
  Rad2Deg/1 -> Coefficients/1(Roll)
  car Aero ApproachVel_1 x/1 -> MATLAB Function/1(Vx), car Aero ApproachVel_1 x_R18/1
  car Aero ApproachVel_1 y/1 -> car Aero ApproachVel_1 y_R18/1, MATLAB Function/2(Vy)
  car Aero ApproachVel_1 z/1 -> car Aero ApproachVel_1 z_R18/1
  car Aero tau_1/1 -> Rad2Deg2/1, car Aero tau_1_R18/1
  Coefficients/1(Coeffs) -> MATLAB Function/3(coeffs)
  MATLAB Function/4(Mx) -> car Aero Trq_1 x_R18/1
  MATLAB Function/1(Fx) -> Drag & DF/1, car Aero Frc_1 x_R18/1
  MATLAB Function/2(Fy) -> car Aero Frc_1 y_R18/1
  Constant/1 -> Coefficients/3(Rideheigth)
  car Aero Frc_1 x/1 -> Terminator/1
  car Aero Frc_1 y/1 -> Terminator1/1
  car Aero Frc_1 z/1 -> Terminator2/1
  car Aero Trq_1 x/1 -> Terminator3/1
  car Aero Trq_1 y/1 -> Terminator4/1
  car Aero Trq_1 z/1 -> Terminator5/1
  MATLAB Function/3(Fz) -> Drag & DF/2, car Aero Frc_1 z_R18/1
  MATLAB Function/5(My) -> Pitch moment/1, car Aero Trq_1 y_R18/1
  MATLAB Function/6(Mz) -> Yaw moment/1, car Aero Trq_1 z_R18/1
  Rad2Deg2/1 -> Coefficients/4(Yaw)

== system TV_2018_HIL/CarMaker/IPG Vehicle3/PowerTrain/Electric Powertrain/E-Gas // E-Motor/Electronic Gas Pedal RL ==
  TC_On : Inport
  VC.Gas : Inport  Port=2
  Define CM Dict : CarMaker4SL/Define CM Dict  xname=E_Gas_RL  xmono=off  xtype=Double4  xdvaplace=None  xnstates=0  xfirststate=0  xinitial=0
  Read CM Dict1 : CarMaker4SL/Read CM Dict  xname=E_Gas_RL  xsync=off
  Read CM Dict2 : CarMaker4SL/Read CM Dict  xname=Car.LongSlipRL  xsync=off
  Subsystem1 : Subsystem
  Switch : Switch
  Write CM Dict : CarMaker4SL/Write CM Dict  xname=E_Gas_RL  xsync=off
  Motor_Gas_RL : Outport
  wires:
  VC.Gas/1 -> Switch/3, Subsystem1/1(VC.Gas)
  Switch/1 -> Motor_Gas_RL/1
  TC_On/1 -> Switch/2
  Subsystem1/1(E_Gas) -> Write CM Dict/1, Switch/1
  Read CM Dict1/1 -> Subsystem1/2(E_Gas.)
  Read CM Dict2/1 -> Subsystem1/3(Car.LongSlip)

== system TV_2018_HIL/CarMaker/IPG Vehicle3/PowerTrain/Electric Powertrain/E-Gas // E-Motor/Electronic Gas Pedal RR ==
  TC_On : Inport
  VC.Gas : Inport  Port=2
  Define CM Dict : CarMaker4SL/Define CM Dict  xname=E_Gas_RR  xmono=off  xtype=Double4  xdvaplace=None  xnstates=0  xfirststate=0  xinitial=0
  Read CM Dict1 : CarMaker4SL/Read CM Dict  xname=E_Gas_RR  xsync=off
  Read CM Dict2 : CarMaker4SL/Read CM Dict  xname=Car.LongSlipRR  xsync=off
  Subsystem1 : Subsystem
  Switch : Switch
  Write CM Dict : CarMaker4SL/Write CM Dict  xname=E_Gas_RR  xsync=off
  Motor_Gas_RR : Outport
  wires:
  TC_On/1 -> Switch/2
  Switch/1 -> Motor_Gas_RR/1
  VC.Gas/1 -> Switch/3, Subsystem1/1(VC.Gas)
  Subsystem1/1(E_Gas) -> Write CM Dict/1, Switch/1
  Read CM Dict2/1 -> Subsystem1/3(Car.LongSlip)
  Read CM Dict1/1 -> Subsystem1/2(E_Gas.)

== system TV_2018_HIL/CarMaker/IPG Vehicle3/PowerTrain/Electric Powertrain/E-Gas // E-Motor/Rotation RL ==
  Gain : Gain  Gain=i_Diff
  Gain1 : Gain  Gain=60/(2*pi)
  Read CM Dict : CarMaker4SL/Read CM Dict  xname=Car.WheelSpd_RL  xsync=off
  Engine_rot_RL : Outport
  wires:
  Read CM Dict/1 -> Gain/1
  Gain/1 -> Gain1/1
  Gain1/1 -> Engine_rot_RL/1

== system TV_2018_HIL/CarMaker/IPG Vehicle3/PowerTrain/Electric Powertrain/E-Gas // E-Motor/Rotation RR ==
  Gain : Gain  Gain=i_Diff
  Gain1 : Gain  Gain=60/(2*pi)
  Read CM Dict : CarMaker4SL/Read CM Dict  xname=Car.WheelSpd_RR  xsync=off
  Engine_rot_RR : Outport
  wires:
  Gain1/1 -> Engine_rot_RR/1
  Gain/1 -> Gain1/1
  Read CM Dict/1 -> Gain/1

== system TV_2018_HIL/CarMaker/Subsystem/Control_System /Slip Rate Control /SMC Traction Control/Slip Rate FL ==
  SR_ref : Inport
  Kp : Inport  Port=2
  SR : Inport  Port=3
  states : Inport  Port=4
  SMC : MATLAB Function  TreatAsAtomicUnit=on
  mu lookup : Lookup_n-D  NumberOfTableDimensions=1  BreakpointsForDimension1="[0  0.15 1]"  Table=[0 1.5 0.75]  ExtrapMethod=Clip  UseLastTableValue=on  InternalRulePriority=Speed  RndMeth=Simplest  InputSameDT=on
  Tc : Outport
  wires:
  SR_ref/1 -> SMC/3(SR_ref)
  SR/1 -> SMC/2(SR), mu lookup/1
  mu lookup/1 -> SMC/1(muOfSlip)
  Kp/1 -> SMC/5(K)
  states/1 -> SMC/4(states)
  SMC/1(TC) -> Tc/1

== system TV_2018_HIL/CarMaker/Subsystem/Control_System /Slip Rate Control /SMC Traction Control/Slip Rate FL1 ==
  SR_ref : Inport
  Kp : Inport  Port=2
  SR : Inport  Port=3
  states : Inport  Port=4
  SMC : MATLAB Function  TreatAsAtomicUnit=on
  mu lookup : Lookup_n-D  NumberOfTableDimensions=1  BreakpointsForDimension1="[0  0.15 1]"  Table=[0 1.5 0.75]  ExtrapMethod=Clip  UseLastTableValue=on  InternalRulePriority=Speed  RndMeth=Simplest  InputSameDT=on
  Tc : Outport
  wires:
  SMC/1(TC) -> Tc/1
  states/1 -> SMC/4(states)
  Kp/1 -> SMC/5(K)
  mu lookup/1 -> SMC/1(muOfSlip)
  SR/1 -> mu lookup/1, SMC/2(SR)
  SR_ref/1 -> SMC/3(SR_ref)

== system TV_2018_HIL/CarMaker/Subsystem/Control_System /Slip Rate Control /SMC Traction Control/Slip Rate FL2 ==
  SR_ref : Inport
  Kp : Inport  Port=2
  SR : Inport  Port=3
  states : Inport  Port=4
  SMC : MATLAB Function  TreatAsAtomicUnit=on
  mu lookup : Lookup_n-D  NumberOfTableDimensions=1  BreakpointsForDimension1="[0  0.15 1]"  Table=[0 1.5 0.75]  ExtrapMethod=Clip  UseLastTableValue=on  InternalRulePriority=Speed  RndMeth=Simplest  InputSameDT=on
  Tc : Outport
  wires:
  SR_ref/1 -> SMC/3(SR_ref)
  SR/1 -> SMC/2(SR), mu lookup/1
  mu lookup/1 -> SMC/1(muOfSlip)
  Kp/1 -> SMC/5(K)
  states/1 -> SMC/4(states)
  SMC/1(TC) -> Tc/1

== system TV_2018_HIL/CarMaker/Subsystem/Control_System /Slip Rate Control /SMC Traction Control/Slip Rate FL3 ==
  SR_ref : Inport
  Kp : Inport  Port=2
  SR : Inport  Port=3
  states : Inport  Port=4
  SMC : MATLAB Function  TreatAsAtomicUnit=on
  mu lookup : Lookup_n-D  NumberOfTableDimensions=1  BreakpointsForDimension1="[0  0.15 1]"  Table=[0 1.5 0.75]  ExtrapMethod=Clip  UseLastTableValue=on  InternalRulePriority=Speed  RndMeth=Simplest  InputSameDT=on
  Tc : Outport
  wires:
  SMC/1(TC) -> Tc/1
  states/1 -> SMC/4(states)
  Kp/1 -> SMC/5(K)
  mu lookup/1 -> SMC/1(muOfSlip)
  SR/1 -> mu lookup/1, SMC/2(SR)
  SR_ref/1 -> SMC/3(SR_ref)

== system TV_2018_HIL/CarMaker/Subsystem/Control_System /Slip Rate Control /Traction Controllers/Slip Rate FL ==
  SR_ref : Inport
  Kp : Inport  Port=2
  Ki : Inport  Port=3
  SR : Inport  Port=4
  Ti_ref : Inport  Port=5
  Constant : Constant  Value=single(0)
  Constant1 : Constant  Value=single(0)
  Discrete-Time Integrator2 : DiscreteIntegrator  ExternalReset=either  InitialConditionSetting=State (most efficient)  SampleTime=-1  ICPrevOutput=DiscIntNeverNeededParam  ICPrevScaledInput=DiscIntNeverNeededParam
  Gain : Gain  Gain=single(-1)
  Gain1 : Gain  Gain=single(-1)
  Gain2 : Gain  Gain=tractionControl.Kb
  Gain7 : Gain  Gain=single(-1)
  Product : Product
  Product1 : Product
  Saturation Dynamic : simulink/Discontinuities/Saturation Dynamic  OutMin=[]  OutMax=[]  OutDataTypeStr=single  OutputDataTypeScalingMode=single  OutDataType=fixdt(1, 16)  OutScaling=2^-10  DoSatur=off
  Saturation Dynamic1 : simulink/Discontinuities/Saturation Dynamic  OutMin=[]  OutMax=[]  OutDataTypeStr=single  OutputDataTypeScalingMode=single  OutDataType=fixdt(1, 16)  OutScaling=2^-10  DoSatur=off
  Sum : Sum  Inputs=|+-
  Sum1 : Sum  Inputs=++|
  Sum2 : Sum  Inputs=|++
  Sum3 : Sum  Inputs=|+-  AccumDataTypeStr=single
  Switch : Switch  Criteria=u2 > Threshold
  Switch1 : Switch  Criteria=u2 > Threshold
  Switch2 : Switch  Criteria=u2 > Threshold
  TC_output : Outport
  wires:
  SR/1 -> Sum/2
  Product/1 -> Sum2/2
  Saturation Dynamic/1 -> Sum2/1, Sum3/1
  Sum/1 -> Product/2, Product1/2
  Gain1/1 -> Switch1/1
  Constant1/1 -> Switch1/3
  Constant/1 -> Switch/1
  Gain/1 -> Switch/3
  Ti_ref/1 -> Discrete-Time Integrator2/2, Switch2/2, Switch1/2, Gain1/1, Gain/1, Switch/2
  SR_ref/1 -> Gain7/1, Switch2/1
  Gain7/1 -> Switch2/3
  Switch2/1 -> Sum/1
  Switch/1 -> Saturation Dynamic1/1, Saturation Dynamic/1
  Switch1/1 -> Saturation Dynamic1/3, Saturation Dynamic/3
  Kp/1 -> Product/1
  Sum1/1 -> Discrete-Time Integrator2/1
  Ki/1 -> Product1/1
  Product1/1 -> Sum1/2
  Discrete-Time Integrator2/1 -> Saturation Dynamic/2, Sum3/2
  Sum3/1 -> Gain2/1
  Gain2/1 -> Sum1/1
  Sum2/1 -> Saturation Dynamic1/2
  Saturation Dynamic1/1 -> TC_output/1

== system TV_2018_HIL/CarMaker/Subsystem/Control_System /Slip Rate Control /Traction Controllers/Slip Rate FR ==
  SR_ref : Inport
  Kp : Inport  Port=2
  Ki : Inport  Port=3
  SR : Inport  Port=4
  Ti_ref : Inport  Port=5
  Constant : Constant  Value=single(0)
  Constant1 : Constant  Value=single(0)
  Discrete-Time Integrator2 : DiscreteIntegrator  ExternalReset=either  InitialConditionSetting=State (most efficient)  SampleTime=-1  ICPrevOutput=DiscIntNeverNeededParam  ICPrevScaledInput=DiscIntNeverNeededParam
  Gain : Gain  Gain=single(-1)
  Gain1 : Gain  Gain=single(-1)
  Gain2 : Gain  Gain=tractionControl.Kb
  Gain7 : Gain  Gain=single(-1)
  PI_Kp 1 : Scope
  PI_Kp 2 : Scope
  PI_Kp 4 : Scope
  Product : Product
  Product1 : Product
  Saturation Dynamic : simulink/Discontinuities/Saturation Dynamic  OutMin=[]  OutMax=[]  OutDataTypeStr=single  OutputDataTypeScalingMode=single  OutDataType=fixdt(1, 16)  OutScaling=2^-10  DoSatur=off
  Saturation Dynamic1 : simulink/Discontinuities/Saturation Dynamic  OutMin=[]  OutMax=[]  OutDataTypeStr=single  OutputDataTypeScalingMode=single  OutDataType=fixdt(1, 16)  OutScaling=2^-10  DoSatur=off
  Sum : Sum  Inputs=|+-
  Sum1 : Sum  Inputs=++|
  Sum2 : Sum  Inputs=|++
  Sum3 : Sum  Inputs=|+-  AccumDataTypeStr=single
  Switch : Switch  Criteria=u2 > Threshold
  Switch1 : Switch  Criteria=u2 > Threshold
  Switch2 : Switch  Criteria=u2 > Threshold
  integrator : Scope
  TC_output : Outport
  wires:
  Saturation Dynamic1/1 -> TC_output/1, PI_Kp 1/1
  Sum2/1 -> Saturation Dynamic1/2
  Gain2/1 -> PI_Kp 4/1, Sum1/1
  Sum3/1 -> Gain2/1
  Discrete-Time Integrator2/1 -> Sum3/2, Saturation Dynamic/2, integrator/1
  Product1/1 -> Sum1/2
  Ki/1 -> Product1/1
  Sum1/1 -> Discrete-Time Integrator2/1
  Kp/1 -> Product/1
  Switch1/1 -> Saturation Dynamic/3, Saturation Dynamic1/3
  Switch/1 -> Saturation Dynamic/1, Saturation Dynamic1/1
  Switch2/1 -> Sum/1
  Gain7/1 -> Switch2/3
  SR_ref/1 -> Switch2/1, Gain7/1
  Ti_ref/1 -> Switch2/2, Discrete-Time Integrator2/2, Switch/2, Gain/1, Gain1/1, Switch1/2
  Gain/1 -> Switch/3
  Constant/1 -> Switch/1
  Constant1/1 -> Switch1/3
  Gain1/1 -> Switch1/1
  Sum/1 -> Product1/2, Product/2
  Saturation Dynamic/1 -> Sum3/1, Sum2/1
  Product/1 -> Sum2/2, PI_Kp 2/1
  SR/1 -> Sum/2

== system TV_2018_HIL/CarMaker/Subsystem/Control_System /Slip Rate Control /Traction Controllers/Slip Rate RL ==
  SR_ref : Inport
  Kp : Inport  Port=2
  Ki : Inport  Port=3
  SR : Inport  Port=4
  Ti_ref : Inport  Port=5
  Constant : Constant  Value=single(0)
  Constant1 : Constant  Value=single(0)
  Discrete-Time Integrator2 : DiscreteIntegrator  ExternalReset=either  InitialConditionSetting=State (most efficient)  SampleTime=-1  ICPrevOutput=DiscIntNeverNeededParam  ICPrevScaledInput=DiscIntNeverNeededParam
  Gain : Gain  Gain=single(-1)
  Gain1 : Gain  Gain=single(-1)
  Gain2 : Gain  Gain=tractionControl.Kb
  Gain7 : Gain  Gain=single(-1)
  PI_Kp 1 : Scope
  PI_Kp 2 : Scope
  PI_Kp 4 : Scope
  Product : Product
  Product1 : Product
  Saturation Dynamic : simulink/Discontinuities/Saturation Dynamic  OutMin=[]  OutMax=[]  OutDataTypeStr=single  OutputDataTypeScalingMode=single  OutDataType=fixdt(1, 16)  OutScaling=2^-10  DoSatur=off
  Saturation Dynamic1 : simulink/Discontinuities/Saturation Dynamic  OutMin=[]  OutMax=[]  OutDataTypeStr=single  OutputDataTypeScalingMode=single  OutDataType=fixdt(1, 16)  OutScaling=2^-10  DoSatur=off
  Sum : Sum  Inputs=|+-
  Sum1 : Sum  Inputs=++|
  Sum2 : Sum  Inputs=|++
  Sum3 : Sum  Inputs=|+-  AccumDataTypeStr=single
  Switch : Switch  Criteria=u2 > Threshold
  Switch1 : Switch  Criteria=u2 > Threshold
  Switch2 : Switch  Criteria=u2 > Threshold
  integrator : Scope
  TC_output : Outport
  wires:
  Saturation Dynamic1/1 -> TC_output/1, PI_Kp 1/1
  Sum2/1 -> Saturation Dynamic1/2
  Gain2/1 -> PI_Kp 4/1, Sum1/1
  Sum3/1 -> Gain2/1
  Discrete-Time Integrator2/1 -> Sum3/2, Saturation Dynamic/2, integrator/1
  Product1/1 -> Sum1/2
  Ki/1 -> Product1/1
  Sum1/1 -> Discrete-Time Integrator2/1
  Kp/1 -> Product/1
  Switch1/1 -> Saturation Dynamic/3, Saturation Dynamic1/3
  Switch/1 -> Saturation Dynamic/1, Saturation Dynamic1/1
  Switch2/1 -> Sum/1
  Gain7/1 -> Switch2/3
  SR_ref/1 -> Switch2/1, Gain7/1
  Ti_ref/1 -> Switch2/2, Discrete-Time Integrator2/2, Switch/2, Gain/1, Gain1/1, Switch1/2
  Gain/1 -> Switch/3
  Constant/1 -> Switch/1
  Constant1/1 -> Switch1/3
  Gain1/1 -> Switch1/1
  Sum/1 -> Product1/2, Product/2
  Saturation Dynamic/1 -> Sum3/1, Sum2/1
  Product/1 -> Sum2/2, PI_Kp 2/1
  SR/1 -> Sum/2

== system TV_2018_HIL/CarMaker/Subsystem/Control_System /Slip Rate Control /Traction Controllers/Slip Rate RR ==
  SR_ref : Inport
  Kp : Inport  Port=2
  Ki : Inport  Port=3
  SR : Inport  Port=4
  Ti_ref : Inport  Port=5
  Constant : Constant  Value=single(0)
  Constant1 : Constant  Value=single(0)
  Discrete-Time Integrator2 : DiscreteIntegrator  ExternalReset=either  InitialConditionSetting=State (most efficient)  SampleTime=-1  ICPrevOutput=DiscIntNeverNeededParam  ICPrevScaledInput=DiscIntNeverNeededParam
  Gain : Gain  Gain=single(-1)
  Gain1 : Gain  Gain=single(-1)
  Gain2 : Gain  Gain=tractionControl.Kb
  Gain7 : Gain  Gain=single(-1)
  PI_Kp 1 : Scope
  PI_Kp 2 : Scope
  PI_Kp 4 : Scope
  Product : Product
  Product1 : Product
  Saturation Dynamic : simulink/Discontinuities/Saturation Dynamic  OutMin=[]  OutMax=[]  OutDataTypeStr=single  OutputDataTypeScalingMode=single  OutDataType=fixdt(1, 16)  OutScaling=2^-10  DoSatur=off
  Saturation Dynamic1 : simulink/Discontinuities/Saturation Dynamic  OutMin=[]  OutMax=[]  OutDataTypeStr=single  OutputDataTypeScalingMode=single  OutDataType=fixdt(1, 16)  OutScaling=2^-10  DoSatur=off
  Sum : Sum  Inputs=|+-
  Sum1 : Sum  Inputs=++|
  Sum2 : Sum  Inputs=|++
  Sum3 : Sum  Inputs=|+-  AccumDataTypeStr=single
  Switch : Switch  Criteria=u2 > Threshold
  Switch1 : Switch  Criteria=u2 > Threshold
  Switch2 : Switch  Criteria=u2 > Threshold
  integrator : Scope
  TC_output : Outport
  wires:
  SR/1 -> Sum/2
  Product/1 -> PI_Kp 2/1, Sum2/2
  Saturation Dynamic/1 -> Sum2/1, Sum3/1
  Sum/1 -> Product/2, Product1/2
  Gain1/1 -> Switch1/1
  Constant1/1 -> Switch1/3
  Constant/1 -> Switch/1
  Gain/1 -> Switch/3
  Ti_ref/1 -> Switch1/2, Gain1/1, Gain/1, Switch/2, Discrete-Time Integrator2/2, Switch2/2
  SR_ref/1 -> Gain7/1, Switch2/1
  Gain7/1 -> Switch2/3
  Switch2/1 -> Sum/1
  Switch/1 -> Saturation Dynamic1/1, Saturation Dynamic/1
  Switch1/1 -> Saturation Dynamic1/3, Saturation Dynamic/3
  Kp/1 -> Product/1
  Sum1/1 -> Discrete-Time Integrator2/1
  Ki/1 -> Product1/1
  Product1/1 -> Sum1/2
  Discrete-Time Integrator2/1 -> integrator/1, Saturation Dynamic/2, Sum3/2
  Sum3/1 -> Gain2/1
  Gain2/1 -> Sum1/1, PI_Kp 4/1
  Sum2/1 -> Saturation Dynamic1/2
  Saturation Dynamic1/1 -> PI_Kp 1/1, TC_output/1

== system TV_2018_HIL/CarMaker/Subsystem/Control_System /Subsystem/2016 adapted/Torque Allocation ==
  T_req : Inport
  states : Inport  Port=2
  maxMotorTorque : Inport  Port=3
  Mz_ref : Inport  Port=4
  Mux1 : Mux  Inputs=3
  Mz : Scope
  Ti_max : Scope
  TorqueAllocation : MATLAB Function  TreatAsAtomicUnit=on
  Ti_lim : Outport
  Mz_allocated : Outport  Port=2
  wires:
  T_req/1 -> TorqueAllocation/1(T_req)
  states/1 -> TorqueAllocation/2(states)
  TorqueAllocation/1(Ti_lim) -> Ti_lim/1
  Mz_ref/1 -> Mux1/3, TorqueAllocation/4(Mz_ref)  "Mz_ref"
  TorqueAllocation/2(Ti_max) -> Ti_max/1
  TorqueAllocation/3(Mz_error) -> Mux1/1  "Mz_error"
  TorqueAllocation/4(Mz_allocated) -> Mux1/2, Mz_allocated/1  "Mz_all"
  Mux1/1 -> Mz/1
  maxMotorTorque/1 -> TorqueAllocation/3(maxMotorTorque)

== system TV_2018_HIL/CarMaker/Subsystem/Control_System /Subsystem/Torque allocation 2016/Torque Allocation ==
  T_req : Inport
  states : Inport  Port=2
  maxMotorTorque : Inport  Port=3
  Mz_ref : Inport  Port=4
  Mux1 : Mux  Inputs=3
  Mz : Scope
  Ti_max : Scope
  TorqueAllocation : MATLAB Function  TreatAsAtomicUnit=on
  Ti_lim : Outport
  Mz_error : Outport  Port=2
  wires:
  T_req/1 -> TorqueAllocation/1(T_req)
  states/1 -> TorqueAllocation/2(states)
  TorqueAllocation/1(Ti_lim) -> Ti_lim/1
  Mz_ref/1 -> Mux1/3, TorqueAllocation/4(Mz_ref)  "Mz_ref"
  TorqueAllocation/2(Ti_max) -> Ti_max/1
  TorqueAllocation/3(Mz_error) -> Mux1/1, Mz_error/1  "Mz_error"
  TorqueAllocation/4(Mz_allocated) -> Mux1/2  "Mz_all"
  Mux1/1 -> Mz/1
  maxMotorTorque/1 -> TorqueAllocation/3(maxMotorTorque)
